simulink model "sFunctionLibrary_WheelTorque_Command_Harness"  (R2025b)
settings: Solver=FixedStepAuto  StartTime=1  StopTime=1000  FixedStep=1  RelTol=1e-3
settings Model: Creator=palla  LastModifiedBy=palla

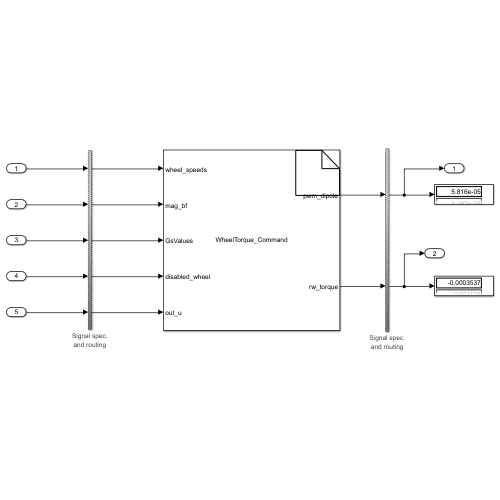
[thumbnail: Simulink's stored preview of the top-level diagram]
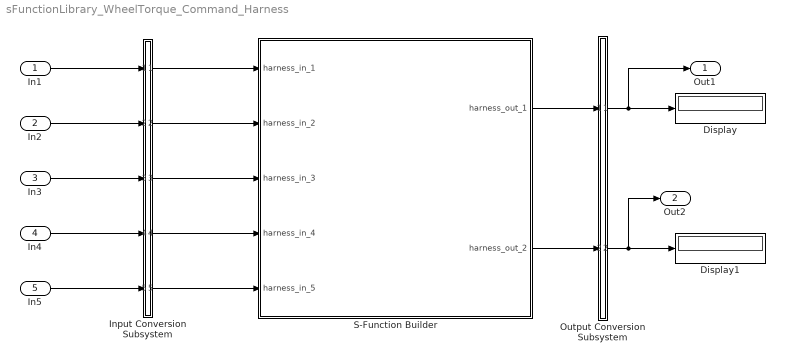
== system sFunctionLibrary_WheelTorque_Command_Harness ==
  In1 : Inport  OutDataTypeStr=single  PortDimensions=[4 1]
  In2 : Inport  Port=2  OutDataTypeStr=single  PortDimensions=[3 1]
  In3 : Inport  Port=3  OutDataTypeStr=single  PortDimensions=[3 4]
  In4 : Inport  Port=4  OutDataTypeStr=int32  PortDimensions=[1 1]
  In5 : Inport  Port=5  OutDataTypeStr=single  PortDimensions=[3 1]
  Display : Display
  Display1 : Display
  Input Conversion Subsystem : Subsystem  Tag=__SLT_ICS__  Description=|
      | Signal spec.
      | and routing
      settings: AttributesFormatString=%<Description>
  Output Conversion Subsystem : Subsystem  Tag=__SLT_OCS__  Description=|
      | Signal spec.
      | and routing
      settings: AttributesFormatString=%<Description>
  S-Function Builder : Subsystem  Tag=__SL_testing_harness_stub_
  Out1 : Outport
  Out2 : Outport  Port=2
  wires:
  Output Conversion Subsystem/1(Outport_1) -> Display/1, Out1/1
  Output Conversion Subsystem/2(Outport_2) -> Display1/1, Out2/1
  Input Conversion Subsystem/1(Outport_1) -> S-Function Builder/1(harness_in_1)
  Input Conversion Subsystem/2(Outport_2) -> S-Function Builder/2(harness_in_2)
  Input Conversion Subsystem/3(Outport_3) -> S-Function Builder/3(harness_in_3)
  Input Conversion Subsystem/4(Outport_4) -> S-Function Builder/4(harness_in_4)
  Input Conversion Subsystem/5(Outport_5) -> S-Function Builder/5(harness_in_5)
  S-Function Builder/1(harness_out_1) -> Output Conversion Subsystem/1(Inport_1)
  S-Function Builder/2(harness_out_2) -> Output Conversion Subsystem/2(Inport_2)
  In1/1 -> Input Conversion Subsystem/1(Inport_1)
  In2/1 -> Input Conversion Subsystem/2(Inport_2)
  In3/1 -> Input Conversion Subsystem/3(Inport_3)
  In4/1 -> Input Conversion Subsystem/4(Inport_4)
  In5/1 -> Input Conversion Subsystem/5(Inport_5)

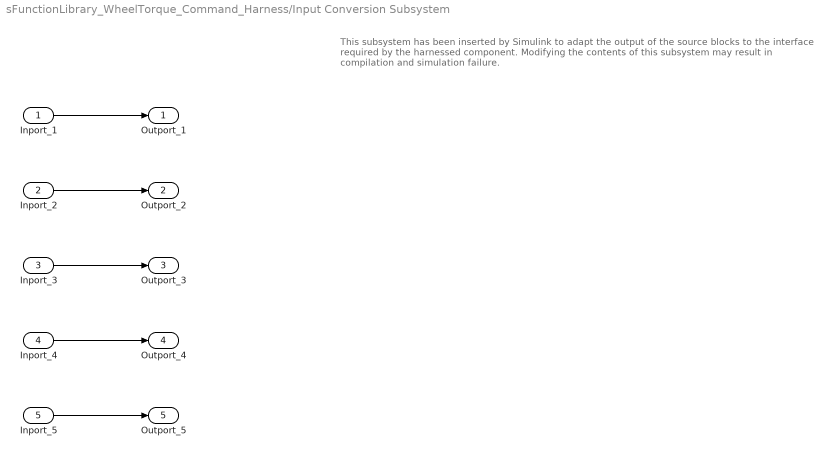
== system sFunctionLibrary_WheelTorque_Command_Harness/Input Conversion Subsystem ==
  note: This subsystem has been inserted by Simulink to adapt the output of the source blocks to the interface required by the harnessed component.
      |  Modifying the contents of this subsystem may result in compilation and simulation failure.
  Inport_1 : Inport
  Inport_2 : Inport  Port=2
  Inport_3 : Inport  Port=3
  Inport_4 : Inport  Port=4
  Inport_5 : Inport  Port=5
  Outport_1 : Outport
  Outport_2 : Outport  Port=2
  Outport_3 : Outport  Port=3
  Outport_4 : Outport  Port=4
  Outport_5 : Outport  Port=5
  wires:
  Inport_1/1 -> Outport_1/1
  Inport_2/1 -> Outport_2/1
  Inport_3/1 -> Outport_3/1
  Inport_4/1 -> Outport_4/1
  Inport_5/1 -> Outport_5/1

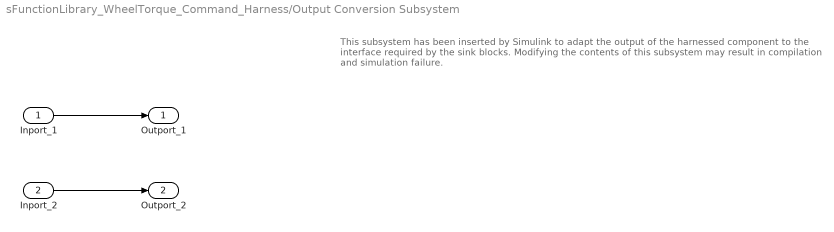
== system sFunctionLibrary_WheelTorque_Command_Harness/Output Conversion Subsystem ==
  note: This subsystem has been inserted by Simulink to adapt the output of the harnessed component to the interface required by the sink blocks.
      |  Modifying the contents of this subsystem may result in compilation and simulation failure.
  Inport_1 : Inport
  Inport_2 : Inport  Port=2
  Outport_1 : Outport
  Outport_2 : Outport  Port=2
  wires:
  Inport_1/1 -> Outport_1/1
  Inport_2/1 -> Outport_2/1

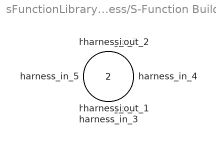
== system sFunctionLibrary_WheelTorque_Command_Harness/S-Function Builder ==
  harness_in_1 : Inport
  harness_in_2 : Inport  Port=2
  harness_in_3 : Inport  Port=3
  harness_in_4 : Inport  Port=4
  harness_in_5 : Inport  Port=5
  harness_out_1 : Outport
  harness_out_2 : Outport  Port=2
